simulink model "ARDRONE_SIM"  (R2014b)
settings: Solver=ode45  StartTime=0.0  StopTime=10  FixedStep=1/400  MaxStep=1  RelTol=1e-3
undefined symbols (not defined in the file or in its folder): X, Y, Z
libraries: sm_lib x204, fl_lib x82, nesl_utility x13, elec_lib x12, simulink x5, aerolibtransform2 x2, aerolibconvert2 x1
(part 2 of 5)

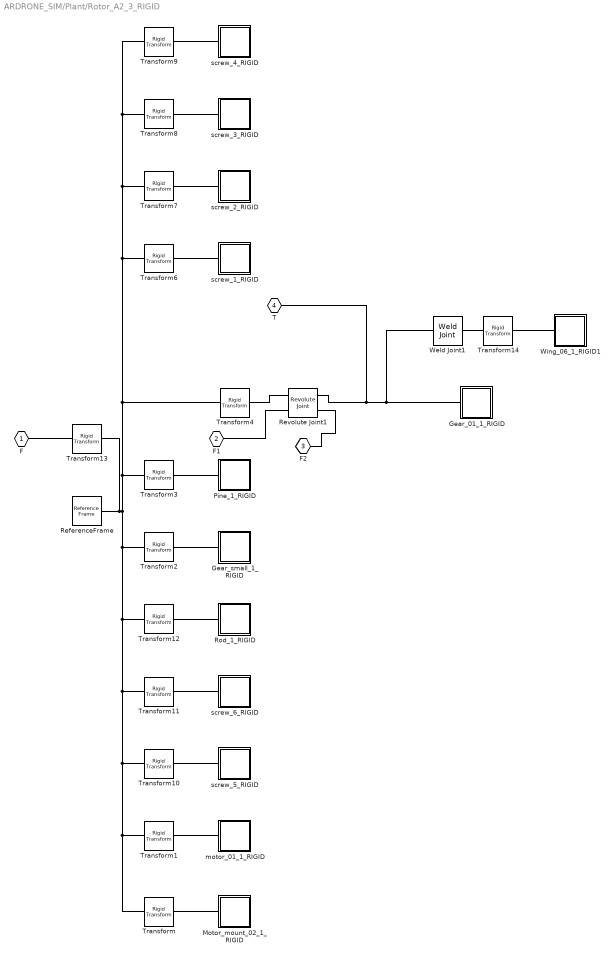
== system ARDRONE_SIM/Plant/Rotor_A2_3_RIGID ==
  Gear_01_1_RIGID : Subsystem
  Gear_small_1_RIGID : Subsystem
  Motor_mount_02_1_RIGID : Subsystem
  Pine_1_RIGID : Subsystem
  ReferenceFrame : sm_lib/Frames and Transforms/Reference Frame  BlockFunction=simmechanics.library.frames_transforms.reference_frame
  Revolute Joint1 : sm_lib/Joints/Revolute Joint  SenseConstraintForce=off  SenseConstraintForceX=off  SenseConstraintForceY=off  SenseConstraintForceZ=off  SenseConstraintTorque=off  SenseConstraintTorqueX=off  SenseConstraintTorqueY=off  SenseConstraintTorqueZ=off  SenseTotalForce=off  SenseTotalForceX=off  SenseTotalForceY=off  SenseTotalForceZ=off  SenseTotalTorque=off  SenseTotalTorqueX=off  SenseTotalTorqueY=off  SenseTotalTorqueZ=off  CompositeWrenchDir=FollowerOnBase  CompositeWrenchFrame=BaseFrame  EquilibriumPosition=0  EquilibriumPositionUnits=deg  SpringStiffness=0  SpringStiffnessUnits=N*m/deg  DampingCoefficient=0  DampingCoefficientUnits=N*m/(deg/s)  TorqueActuationMode=InputTorque  MotionActuationMode=ComputedMotion  SensePosition=off  SenseVelocity=on  SenseAcceleration=off  SenseTorqueForce=off  PositionTargetValue=0  PositionTargetValueUnits=deg  PositionTargetSpecify=off  PositionTargetPriority=High  VelocityTargetValue=500  VelocityTargetValueUnits=deg/s  VelocityTargetSpecify=off  VelocityTargetPriority=High  BlockFunction=simmechanics.library.joints.revolute_joint
  Rod_1_RIGID : Subsystem
  Transform : sm_lib/Frames and Transforms/Rigid Transform  TranslationMethod=None  TranslationLengthUnit=m  TranslationStandardAxis=+Z  TranslationStandardOffset=0  TranslationCartesianOffset=[0 0 0]  TranslationROffset=0  TranslationROffsetUnits=m  TranslationZOffset=0  TranslationZOffsetUnits=m  TranslationThetaOffset=0  TranslationThetaOffsetUnits=deg  RotationMethod=None  RotationAngleUnits=deg  RotationStandardAxis=+Z  RotationAngle=0  RotationArbitraryAxis=[0 0 1]  FollAlignAxisA=+X  BaseAlignAxisA=+Y  FollAlignAxisB=+Y  BaseAlignAxisB=+Z  RotationMatrix=[1 0 0; 0 1 0; 0 0 1]  BlockFunction=simmechanics.library.frames_transforms.rigid_transform
  Transform1 : sm_lib/Frames and Transforms/Rigid Transform  TranslationMethod=Cartesian  TranslationLengthUnit=mm  TranslationStandardAxis=+Z  TranslationStandardOffset=0  TranslationCartesianOffset=[3.1499999999999999 0 -20.598100000000002]  TranslationROffset=0  TranslationROffsetUnits=m  TranslationZOffset=0  TranslationZOffsetUnits=m  TranslationThetaOffset=0  TranslationThetaOffsetUnits=deg  RotationMethod=ArbitraryAxis  RotationAngleUnits=rad  RotationStandardAxis=+Z  RotationAngle=3.1403990331346985  RotationArbitraryAxis=[0 0 1]  FollAlignAxisA=+X  BaseAlignAxisA=+Y  FollAlignAxisB=+Y  BaseAlignAxisB=+Z  RotationMatrix=[1 0 0; 0 1 0; 0 0 1]  BlockFunction=simmechanics.library.frames_transforms.rigid_transform
  Transform10 : sm_lib/Frames and Transforms/Rigid Transform  TranslationMethod=Cartesian  TranslationLengthUnit=mm  TranslationStandardAxis=+Z  TranslationStandardOffset=0  TranslationCartesianOffset=[-19.174799999999998 6.3336399999999999 -3.4415300000000002]  TranslationROffset=0  TranslationROffsetUnits=m  TranslationZOffset=0  TranslationZOffsetUnits=m  TranslationThetaOffset=0  TranslationThetaOffsetUnits=deg  RotationMethod=ArbitraryAxis  RotationAngleUnits=rad  RotationStandardAxis=+Z  RotationAngle=1.5707963267948968  RotationArbitraryAxis=[0 1 0]  FollAlignAxisA=+X  BaseAlignAxisA=+Y  FollAlignAxisB=+Y  BaseAlignAxisB=+Z  RotationMatrix=[1 0 0; 0 1 0; 0 0 1]  BlockFunction=simmechanics.library.frames_transforms.rigid_transform
  Transform11 : sm_lib/Frames and Transforms/Rigid Transform  TranslationMethod=Cartesian  TranslationLengthUnit=mm  TranslationStandardAxis=+Z  TranslationStandardOffset=0  TranslationCartesianOffset=[21.5288 3.5415400000000004 -3.4415300000000002]  TranslationROffset=0  TranslationROffsetUnits=m  TranslationZOffset=0  TranslationZOffsetUnits=m  TranslationThetaOffset=0  TranslationThetaOffsetUnits=deg  RotationMethod=ArbitraryAxis  RotationAngleUnits=rad  RotationStandardAxis=+Z  RotationAngle=1.5707963267948968  RotationArbitraryAxis=[0 1 0]  FollAlignAxisA=+X  BaseAlignAxisA=+Y  FollAlignAxisB=+Y  BaseAlignAxisB=+Z  RotationMatrix=[1 0 0; 0 1 0; 0 0 1]  BlockFunction=simmechanics.library.frames_transforms.rigid_transform
  Transform12 : sm_lib/Frames and Transforms/Rigid Transform  TranslationMethod=Cartesian  TranslationLengthUnit=mm  TranslationStandardAxis=+Z  TranslationStandardOffset=0  TranslationCartesianOffset=[-18.649999999999999 0.033281699999999997 4.0656299999999996]  TranslationROffset=0  TranslationROffsetUnits=m  TranslationZOffset=0  TranslationZOffsetUnits=m  TranslationThetaOffset=0  TranslationThetaOffsetUnits=deg  RotationMethod=ArbitraryAxis  RotationAngleUnits=rad  RotationStandardAxis=+Z  RotationAngle=2.0943951023931953  RotationArbitraryAxis=[0.57735026918962584 -0.57735026918962584 -0.57735026918962584]  FollAlignAxisA=+X  BaseAlignAxisA=+Y  FollAlignAxisB=+Y  BaseAlignAxisB=+Z  RotationMatrix=[1 0 0; 0 1 0; 0 0 1]  BlockFunction=simmechanics.library.frames_transforms.rigid_transform
  Transform13 : sm_lib/Frames and Transforms/Rigid Transform  TranslationMethod=Cartesian  TranslationLengthUnit=mm  TranslationStandardAxis=+Z  TranslationStandardOffset=0  TranslationCartesianOffset=[0.036458000000000004 158.29999999999998 -8.3114100000000004]  TranslationROffset=0  TranslationROffsetUnits=m  TranslationZOffset=0  TranslationZOffsetUnits=m  TranslationThetaOffset=0  TranslationThetaOffsetUnits=deg  RotationMethod=ArbitraryAxis  RotationAngleUnits=rad  RotationStandardAxis=+Z  RotationAngle=1.5707964793812017  RotationArbitraryAxis=[-0.00039062294039628431 -0.00039062294039628431 0.99999984741370684]  FollAlignAxisA=+X  BaseAlignAxisA=+Y  FollAlignAxisB=+Y  BaseAlignAxisB=+Z  RotationMatrix=[1 0 0; 0 1 0; 0 0 1]  BlockFunction=simmechanics.library.frames_transforms.rigid_transform
  Transform14 : sm_lib/Frames and Transforms/Rigid Transform  TranslationMethod=Cartesian  TranslationLengthUnit=mm  TranslationStandardAxis=+Z  TranslationStandardOffset=0  TranslationCartesianOffset=[-93.759200000000007+14 -6.75 19]  TranslationROffset=0  TranslationROffsetUnits=m  TranslationZOffset=0  TranslationZOffsetUnits=m  TranslationThetaOffset=0  TranslationThetaOffsetUnits=deg  RotationMethod=None  RotationAngleUnits=rad  RotationStandardAxis=+Z  RotationAngle=2.5698479866285431  RotationArbitraryAxis=[0 0 1]  FollAlignAxisA=+X  BaseAlignAxisA=+Y  FollAlignAxisB=+Y  BaseAlignAxisB=+Z  RotationMatrix=[1 0 0; 0 1 0; 0 0 1]  BlockFunction=simmechanics.library.frames_transforms.rigid_transform
  Transform2 : sm_lib/Frames and Transforms/Rigid Transform  TranslationMethod=Cartesian  TranslationLengthUnit=mm  TranslationStandardAxis=+Z  TranslationStandardOffset=0  TranslationCartesianOffset=[3.1499999999999999 0 16.5459]  TranslationROffset=0  TranslationROffsetUnits=m  TranslationZOffset=0  TranslationZOffsetUnits=m  TranslationThetaOffset=0  TranslationThetaOffsetUnits=deg  RotationMethod=ArbitraryAxis  RotationAngleUnits=rad  RotationStandardAxis=+Z  RotationAngle=2.5767486738905112  RotationArbitraryAxis=[0 0 1]  FollAlignAxisA=+X  BaseAlignAxisA=+Y  FollAlignAxisB=+Y  BaseAlignAxisB=+Z  RotationMatrix=[1 0 0; 0 1 0; 0 0 1]  BlockFunction=simmechanics.library.frames_transforms.rigid_transform
  Transform3 : sm_lib/Frames and Transforms/Rigid Transform  TranslationMethod=Cartesian  TranslationLengthUnit=mm  TranslationStandardAxis=+Z  TranslationStandardOffset=0  TranslationCartesianOffset=[23.150000000000002 0 16.899999999999999]  TranslationROffset=0  TranslationROffsetUnits=m  TranslationZOffset=0  TranslationZOffsetUnits=m  TranslationThetaOffset=0  TranslationThetaOffsetUnits=deg  RotationMethod=ArbitraryAxis  RotationAngleUnits=rad  RotationStandardAxis=+Z  RotationAngle=3.1415926535897931  RotationArbitraryAxis=[0.94291276431253201 0.33303981578258707 0]  FollAlignAxisA=+X  BaseAlignAxisA=+Y  FollAlignAxisB=+Y  BaseAlignAxisB=+Z  RotationMatrix=[1 0 0; 0 1 0; 0 0 1]  BlockFunction=simmechanics.library.frames_transforms.rigid_transform
  Transform4 : sm_lib/Frames and Transforms/Rigid Transform  TranslationMethod=Cartesian  TranslationLengthUnit=mm  TranslationStandardAxis=+Z  TranslationStandardOffset=0  TranslationCartesianOffset=[23.150000000000002 0 15.25]  TranslationROffset=0  TranslationROffsetUnits=m  TranslationZOffset=0  TranslationZOffsetUnits=m  TranslationThetaOffset=0  TranslationThetaOffsetUnits=deg  RotationMethod=ArbitraryAxis  RotationAngleUnits=rad  RotationStandardAxis=+Z  RotationAngle=2.5698479866285431  RotationArbitraryAxis=[0 0 1]  FollAlignAxisA=+X  BaseAlignAxisA=+Y  FollAlignAxisB=+Y  BaseAlignAxisB=+Z  RotationMatrix=[1 0 0; 0 1 0; 0 0 1]  BlockFunction=simmechanics.library.frames_transforms.rigid_transform
  Transform6 : sm_lib/Frames and Transforms/Rigid Transform  TranslationMethod=Cartesian  TranslationLengthUnit=mm  TranslationStandardAxis=+Z  TranslationStandardOffset=0  TranslationCartesianOffset=[0.86552300000000004 3.8769999999999998 8.9434500000000003]  TranslationROffset=0  TranslationROffsetUnits=m  TranslationZOffset=0  TranslationZOffsetUnits=m  TranslationThetaOffset=0  TranslationThetaOffsetUnits=deg  RotationMethod=ArbitraryAxis  RotationAngleUnits=rad  RotationStandardAxis=+Z  RotationAngle=1.6089415653150072  RotationArbitraryAxis=[0.19166392654548023 -0.96256422046652934 0.19166392654548023]  FollAlignAxisA=+X  BaseAlignAxisA=+Y  FollAlignAxisB=+Y  BaseAlignAxisB=+Z  RotationMatrix=[1 0 0; 0 1 0; 0 0 1]  BlockFunction=simmechanics.library.frames_transforms.rigid_transform
  Transform7 : sm_lib/Frames and Transforms/Rigid Transform  TranslationMethod=Cartesian  TranslationLengthUnit=mm  TranslationStandardAxis=+Z  TranslationStandardOffset=0  TranslationCartesianOffset=[0.9346540000000001 -3.9169199999999997 8.9434500000000003]  TranslationROffset=0  TranslationROffsetUnits=m  TranslationZOffset=0  TranslationZOffsetUnits=m  TranslationThetaOffset=0  TranslationThetaOffsetUnits=deg  RotationMethod=ArbitraryAxis  RotationAngleUnits=rad  RotationStandardAxis=+Z  RotationAngle=1.5707963267948968  RotationArbitraryAxis=[-0 -1 -0]  FollAlignAxisA=+X  BaseAlignAxisA=+Y  FollAlignAxisB=+Y  BaseAlignAxisB=+Z  RotationMatrix=[1 0 0; 0 1 0; 0 0 1]  BlockFunction=simmechanics.library.frames_transforms.rigid_transform
  Transform8 : sm_lib/Frames and Transforms/Rigid Transform  TranslationMethod=Cartesian  TranslationLengthUnit=mm  TranslationStandardAxis=+Z  TranslationStandardOffset=0  TranslationCartesianOffset=[7.6498200000000001 0.0399131 8.9434500000000003]  TranslationROffset=0  TranslationROffsetUnits=m  TranslationZOffset=0  TranslationZOffsetUnits=m  TranslationThetaOffset=0  TranslationThetaOffsetUnits=deg  RotationMethod=ArbitraryAxis  RotationAngleUnits=rad  RotationStandardAxis=+Z  RotationAngle=1.5707963267948968  RotationArbitraryAxis=[-0 -1 -0]  FollAlignAxisA=+X  BaseAlignAxisA=+Y  FollAlignAxisB=+Y  BaseAlignAxisB=+Z  RotationMatrix=[1 0 0; 0 1 0; 0 0 1]  BlockFunction=simmechanics.library.frames_transforms.rigid_transform
  Transform9 : sm_lib/Frames and Transforms/Rigid Transform  TranslationMethod=Cartesian  TranslationLengthUnit=mm  TranslationStandardAxis=+Z  TranslationStandardOffset=0  TranslationCartesianOffset=[-19.420099999999998 -6.4385499999999993 -3.4415300000000002]  TranslationROffset=0  TranslationROffsetUnits=m  TranslationZOffset=0  TranslationZOffsetUnits=m  TranslationThetaOffset=0  TranslationThetaOffsetUnits=deg  RotationMethod=ArbitraryAxis  RotationAngleUnits=rad  RotationStandardAxis=+Z  RotationAngle=1.5707963267948968  RotationArbitraryAxis=[0 1 0]  FollAlignAxisA=+X  BaseAlignAxisA=+Y  FollAlignAxisB=+Y  BaseAlignAxisB=+Z  RotationMatrix=[1 0 0; 0 1 0; 0 0 1]  BlockFunction=simmechanics.library.frames_transforms.rigid_transform
  Weld Joint1 : sm_lib/Joints/Weld Joint  SenseConstraintForce=off  SenseConstraintForceX=off  SenseConstraintForceY=off  SenseConstraintForceZ=off  SenseConstraintTorque=off  SenseConstraintTorqueX=off  SenseConstraintTorqueY=off  SenseConstraintTorqueZ=off  SenseTotalForce=off  SenseTotalForceX=off  SenseTotalForceY=off  SenseTotalForceZ=off  SenseTotalTorque=off  SenseTotalTorqueX=off  SenseTotalTorqueY=off  SenseTotalTorqueZ=off  CompositeWrenchDir=FollowerOnBase  CompositeWrenchFrame=BaseFrame  BlockFunction=simmechanics.library.joints.weld_joint
  Wing_06_1_RIGID1 : Subsystem
  motor_01_1_RIGID : Subsystem
  screw_1_RIGID : Subsystem
  screw_2_RIGID : Subsystem
  screw_3_RIGID : Subsystem
  screw_4_RIGID : Subsystem
  screw_5_RIGID : Subsystem
  screw_6_RIGID : Subsystem
  F : PMIOPort  Port=1  Side=Left
  F1 : PMIOPort  Port=2  Side=Right
  F2 : PMIOPort  Port=3  Side=Left
  T : PMIOPort  Port=4  Side=Right
  connections:
  Motor_mount_02_1_RIGID/LConn1 -- Transform/RConn1
  Transform1/RConn1 -- motor_01_1_RIGID/LConn1
  Transform10/RConn1 -- screw_5_RIGID/LConn1
  Transform11/RConn1 -- screw_6_RIGID/LConn1
  Rod_1_RIGID/LConn1 -- Transform12/RConn1
  Transform13/LConn1 -- F/RConn1
  Gear_small_1_RIGID/LConn1 -- Transform2/RConn1
  Pine_1_RIGID/LConn1 -- Transform3/RConn1
  Transform6/RConn1 -- screw_1_RIGID/LConn1
  Transform7/RConn1 -- screw_2_RIGID/LConn1
  Transform8/RConn1 -- screw_3_RIGID/LConn1
  Transform9/RConn1 -- screw_4_RIGID/LConn1
  Weld Joint1/LConn1 -- T/RConn1 -- Revolute Joint1/RConn1 -- Gear_01_1_RIGID/LConn1
  Transform14/RConn1 -- Wing_06_1_RIGID1/LConn1
  Transform/LConn1 -- Transform4/LConn1 -- Transform8/LConn1 -- Transform9/LConn1 -- Transform7/LConn1 -- Transform6/LConn1 -- Transform3/LConn1 -- ReferenceFrame/RConn1 -- Transform13/RConn1 -- Transform2/LConn1 -- Transform12/LConn1 -- Transform11/LConn1 -- Transform10/LConn1 -- Transform1/LConn1
  Transform14/LConn1 -- Weld Joint1/RConn1
  Transform4/RConn1 -- Revolute Joint1/LConn1
  F1/RConn1 -- Revolute Joint1/LConn2
  F2/RConn1 -- Revolute Joint1/RConn2

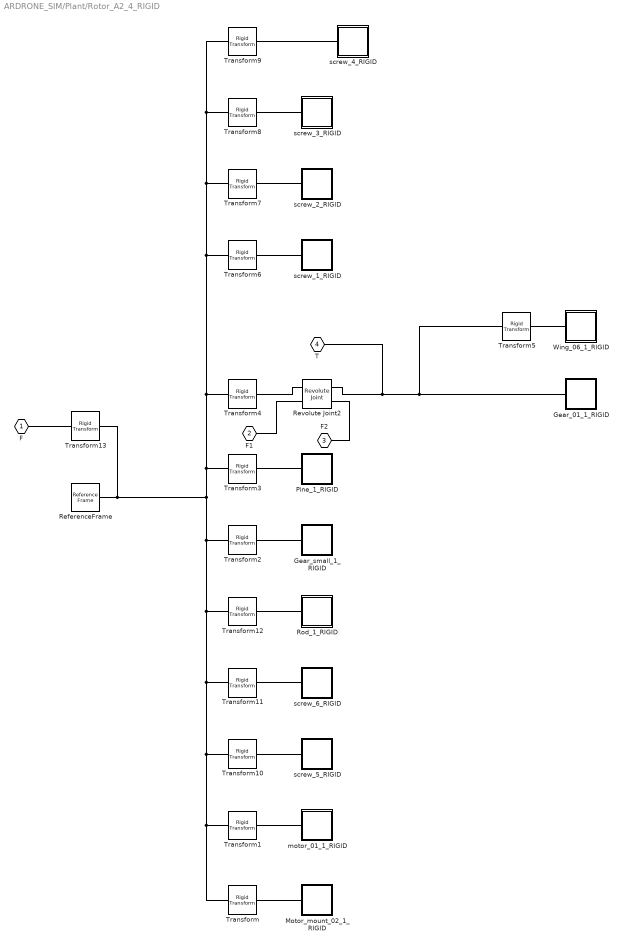
== system ARDRONE_SIM/Plant/Rotor_A2_4_RIGID ==
  Gear_01_1_RIGID : Subsystem
  Gear_small_1_RIGID : Subsystem
  Motor_mount_02_1_RIGID : Subsystem
  Pine_1_RIGID : Subsystem
  ReferenceFrame : sm_lib/Frames and Transforms/Reference Frame  BlockFunction=simmechanics.library.frames_transforms.reference_frame
  Revolute Joint2 : sm_lib/Joints/Revolute Joint  SenseConstraintForce=off  SenseConstraintForceX=off  SenseConstraintForceY=off  SenseConstraintForceZ=off  SenseConstraintTorque=off  SenseConstraintTorqueX=off  SenseConstraintTorqueY=off  SenseConstraintTorqueZ=off  SenseTotalForce=off  SenseTotalForceX=off  SenseTotalForceY=off  SenseTotalForceZ=off  SenseTotalTorque=off  SenseTotalTorqueX=off  SenseTotalTorqueY=off  SenseTotalTorqueZ=off  CompositeWrenchDir=FollowerOnBase  CompositeWrenchFrame=BaseFrame  EquilibriumPosition=0  EquilibriumPositionUnits=deg  SpringStiffness=0  SpringStiffnessUnits=N*m/deg  DampingCoefficient=0  DampingCoefficientUnits=N*m/(deg/s)  TorqueActuationMode=InputTorque  MotionActuationMode=ComputedMotion  SensePosition=off  SenseVelocity=on  SenseAcceleration=off  SenseTorqueForce=off  PositionTargetValue=0  PositionTargetValueUnits=deg  PositionTargetSpecify=off  PositionTargetPriority=High  VelocityTargetValue=500  VelocityTargetValueUnits=deg/s  VelocityTargetSpecify=off  VelocityTargetPriority=High  BlockFunction=simmechanics.library.joints.revolute_joint
  Rod_1_RIGID : Subsystem
  Transform : sm_lib/Frames and Transforms/Rigid Transform  TranslationMethod=None  TranslationLengthUnit=m  TranslationStandardAxis=+Z  TranslationStandardOffset=0  TranslationCartesianOffset=[0 0 0]  TranslationROffset=0  TranslationROffsetUnits=m  TranslationZOffset=0  TranslationZOffsetUnits=m  TranslationThetaOffset=0  TranslationThetaOffsetUnits=deg  RotationMethod=None  RotationAngleUnits=deg  RotationStandardAxis=+Z  RotationAngle=0  RotationArbitraryAxis=[0 0 1]  FollAlignAxisA=+X  BaseAlignAxisA=+Y  FollAlignAxisB=+Y  BaseAlignAxisB=+Z  RotationMatrix=[1 0 0; 0 1 0; 0 0 1]  BlockFunction=simmechanics.library.frames_transforms.rigid_transform
  Transform1 : sm_lib/Frames and Transforms/Rigid Transform  TranslationMethod=Cartesian  TranslationLengthUnit=mm  TranslationStandardAxis=+Z  TranslationStandardOffset=0  TranslationCartesianOffset=[3.1499999999999999 0 -20.598100000000002]  TranslationROffset=0  TranslationROffsetUnits=m  TranslationZOffset=0  TranslationZOffsetUnits=m  TranslationThetaOffset=0  TranslationThetaOffsetUnits=deg  RotationMethod=ArbitraryAxis  RotationAngleUnits=rad  RotationStandardAxis=+Z  RotationAngle=3.1403990331346985  RotationArbitraryAxis=[0 0 1]  FollAlignAxisA=+X  BaseAlignAxisA=+Y  FollAlignAxisB=+Y  BaseAlignAxisB=+Z  RotationMatrix=[1 0 0; 0 1 0; 0 0 1]  BlockFunction=simmechanics.library.frames_transforms.rigid_transform
  Transform10 : sm_lib/Frames and Transforms/Rigid Transform  TranslationMethod=Cartesian  TranslationLengthUnit=mm  TranslationStandardAxis=+Z  TranslationStandardOffset=0  TranslationCartesianOffset=[-19.174799999999998 6.3336399999999999 -3.4415300000000002]  TranslationROffset=0  TranslationROffsetUnits=m  TranslationZOffset=0  TranslationZOffsetUnits=m  TranslationThetaOffset=0  TranslationThetaOffsetUnits=deg  RotationMethod=ArbitraryAxis  RotationAngleUnits=rad  RotationStandardAxis=+Z  RotationAngle=1.5707963267948968  RotationArbitraryAxis=[0 1 0]  FollAlignAxisA=+X  BaseAlignAxisA=+Y  FollAlignAxisB=+Y  BaseAlignAxisB=+Z  RotationMatrix=[1 0 0; 0 1 0; 0 0 1]  BlockFunction=simmechanics.library.frames_transforms.rigid_transform
  Transform11 : sm_lib/Frames and Transforms/Rigid Transform  TranslationMethod=Cartesian  TranslationLengthUnit=mm  TranslationStandardAxis=+Z  TranslationStandardOffset=0  TranslationCartesianOffset=[21.5288 3.5415400000000004 -3.4415300000000002]  TranslationROffset=0  TranslationROffsetUnits=m  TranslationZOffset=0  TranslationZOffsetUnits=m  TranslationThetaOffset=0  TranslationThetaOffsetUnits=deg  RotationMethod=ArbitraryAxis  RotationAngleUnits=rad  RotationStandardAxis=+Z  RotationAngle=1.5707963267948968  RotationArbitraryAxis=[0 1 0]  FollAlignAxisA=+X  BaseAlignAxisA=+Y  FollAlignAxisB=+Y  BaseAlignAxisB=+Z  RotationMatrix=[1 0 0; 0 1 0; 0 0 1]  BlockFunction=simmechanics.library.frames_transforms.rigid_transform
  Transform12 : sm_lib/Frames and Transforms/Rigid Transform  TranslationMethod=Cartesian  TranslationLengthUnit=mm  TranslationStandardAxis=+Z  TranslationStandardOffset=0  TranslationCartesianOffset=[-18.649999999999999 0.033281699999999997 4.0656299999999996]  TranslationROffset=0  TranslationROffsetUnits=m  TranslationZOffset=0  TranslationZOffsetUnits=m  TranslationThetaOffset=0  TranslationThetaOffsetUnits=deg  RotationMethod=ArbitraryAxis  RotationAngleUnits=rad  RotationStandardAxis=+Z  RotationAngle=2.0943951023931953  RotationArbitraryAxis=[0.57735026918962584 -0.57735026918962584 -0.57735026918962584]  FollAlignAxisA=+X  BaseAlignAxisA=+Y  FollAlignAxisB=+Y  BaseAlignAxisB=+Z  RotationMatrix=[1 0 0; 0 1 0; 0 0 1]  BlockFunction=simmechanics.library.frames_transforms.rigid_transform
  Transform13 : sm_lib/Frames and Transforms/Rigid Transform  TranslationMethod=Cartesian  TranslationLengthUnit=mm  TranslationStandardAxis=+Z  TranslationStandardOffset=0  TranslationCartesianOffset=[158.29999999999998 -0.037259299999999995 -8.3156300000000005]  TranslationROffset=0  TranslationROffsetUnits=m  TranslationZOffset=0  TranslationZOffsetUnits=m  TranslationThetaOffset=0  TranslationThetaOffsetUnits=deg  RotationMethod=None  RotationAngleUnits=deg  RotationStandardAxis=+Z  RotationAngle=0  RotationArbitraryAxis=[0 0 1]  FollAlignAxisA=+X  BaseAlignAxisA=+Y  FollAlignAxisB=+Y  BaseAlignAxisB=+Z  RotationMatrix=[1 0 0; 0 1 0; 0 0 1]  BlockFunction=simmechanics.library.frames_transforms.rigid_transform
  Transform2 : sm_lib/Frames and Transforms/Rigid Transform  TranslationMethod=Cartesian  TranslationLengthUnit=mm  TranslationStandardAxis=+Z  TranslationStandardOffset=0  TranslationCartesianOffset=[3.1499999999999999 0 16.5459]  TranslationROffset=0  TranslationROffsetUnits=m  TranslationZOffset=0  TranslationZOffsetUnits=m  TranslationThetaOffset=0  TranslationThetaOffsetUnits=deg  RotationMethod=ArbitraryAxis  RotationAngleUnits=rad  RotationStandardAxis=+Z  RotationAngle=2.5767486738905112  RotationArbitraryAxis=[0 0 1]  FollAlignAxisA=+X  BaseAlignAxisA=+Y  FollAlignAxisB=+Y  BaseAlignAxisB=+Z  RotationMatrix=[1 0 0; 0 1 0; 0 0 1]  BlockFunction=simmechanics.library.frames_transforms.rigid_transform
  Transform3 : sm_lib/Frames and Transforms/Rigid Transform  TranslationMethod=Cartesian  TranslationLengthUnit=mm  TranslationStandardAxis=+Z  TranslationStandardOffset=0  TranslationCartesianOffset=[23.150000000000002 0 16.899999999999999]  TranslationROffset=0  TranslationROffsetUnits=m  TranslationZOffset=0  TranslationZOffsetUnits=m  TranslationThetaOffset=0  TranslationThetaOffsetUnits=deg  RotationMethod=ArbitraryAxis  RotationAngleUnits=rad  RotationStandardAxis=+Z  RotationAngle=3.1415926535897931  RotationArbitraryAxis=[0.94291276431253201 0.33303981578258707 0]  FollAlignAxisA=+X  BaseAlignAxisA=+Y  FollAlignAxisB=+Y  BaseAlignAxisB=+Z  RotationMatrix=[1 0 0; 0 1 0; 0 0 1]  BlockFunction=simmechanics.library.frames_transforms.rigid_transform
  Transform4 : sm_lib/Frames and Transforms/Rigid Transform  TranslationMethod=Cartesian  TranslationLengthUnit=mm  TranslationStandardAxis=+Z  TranslationStandardOffset=0  TranslationCartesianOffset=[23.150000000000002 0 15.25]  TranslationROffset=0  TranslationROffsetUnits=m  TranslationZOffset=0  TranslationZOffsetUnits=m  TranslationThetaOffset=0  TranslationThetaOffsetUnits=deg  RotationMethod=ArbitraryAxis  RotationAngleUnits=rad  RotationStandardAxis=+Z  RotationAngle=2.5698479866285431  RotationArbitraryAxis=[0 0 1]  FollAlignAxisA=+X  BaseAlignAxisA=+Y  FollAlignAxisB=+Y  BaseAlignAxisB=+Z  RotationMatrix=[1 0 0; 0 1 0; 0 0 1]  BlockFunction=simmechanics.library.frames_transforms.rigid_transform
  Transform5 : sm_lib/Frames and Transforms/Rigid Transform  TranslationMethod=Cartesian  TranslationLengthUnit=mm  TranslationStandardAxis=+Z  TranslationStandardOffset=0  TranslationCartesianOffset=[-93.759200000000007+14 -6.75 19]  TranslationROffset=0  TranslationROffsetUnits=m  TranslationZOffset=0  TranslationZOffsetUnits=m  TranslationThetaOffset=0  TranslationThetaOffsetUnits=deg  RotationMethod=None  RotationAngleUnits=rad  RotationStandardAxis=+Z  RotationAngle=2.5698479866285431  RotationArbitraryAxis=[0 0 1]  FollAlignAxisA=+X  BaseAlignAxisA=+Y  FollAlignAxisB=+Y  BaseAlignAxisB=+Z  RotationMatrix=[1 0 0; 0 1 0; 0 0 1]  BlockFunction=simmechanics.library.frames_transforms.rigid_transform
  Transform6 : sm_lib/Frames and Transforms/Rigid Transform  TranslationMethod=Cartesian  TranslationLengthUnit=mm  TranslationStandardAxis=+Z  TranslationStandardOffset=0  TranslationCartesianOffset=[0.86552300000000004 3.8769999999999998 8.9434500000000003]  TranslationROffset=0  TranslationROffsetUnits=m  TranslationZOffset=0  TranslationZOffsetUnits=m  TranslationThetaOffset=0  TranslationThetaOffsetUnits=deg  RotationMethod=ArbitraryAxis  RotationAngleUnits=rad  RotationStandardAxis=+Z  RotationAngle=1.6089415653150072  RotationArbitraryAxis=[0.19166392654548023 -0.96256422046652934 0.19166392654548023]  FollAlignAxisA=+X  BaseAlignAxisA=+Y  FollAlignAxisB=+Y  BaseAlignAxisB=+Z  RotationMatrix=[1 0 0; 0 1 0; 0 0 1]  BlockFunction=simmechanics.library.frames_transforms.rigid_transform
  Transform7 : sm_lib/Frames and Transforms/Rigid Transform  TranslationMethod=Cartesian  TranslationLengthUnit=mm  TranslationStandardAxis=+Z  TranslationStandardOffset=0  TranslationCartesianOffset=[0.9346540000000001 -3.9169199999999997 8.9434500000000003]  TranslationROffset=0  TranslationROffsetUnits=m  TranslationZOffset=0  TranslationZOffsetUnits=m  TranslationThetaOffset=0  TranslationThetaOffsetUnits=deg  RotationMethod=ArbitraryAxis  RotationAngleUnits=rad  RotationStandardAxis=+Z  RotationAngle=1.5707963267948968  RotationArbitraryAxis=[-0 -1 -0]  FollAlignAxisA=+X  BaseAlignAxisA=+Y  FollAlignAxisB=+Y  BaseAlignAxisB=+Z  RotationMatrix=[1 0 0; 0 1 0; 0 0 1]  BlockFunction=simmechanics.library.frames_transforms.rigid_transform
  Transform8 : sm_lib/Frames and Transforms/Rigid Transform  TranslationMethod=Cartesian  TranslationLengthUnit=mm  TranslationStandardAxis=+Z  TranslationStandardOffset=0  TranslationCartesianOffset=[7.6498200000000001 0.0399131 8.9434500000000003]  TranslationROffset=0  TranslationROffsetUnits=m  TranslationZOffset=0  TranslationZOffsetUnits=m  TranslationThetaOffset=0  TranslationThetaOffsetUnits=deg  RotationMethod=ArbitraryAxis  RotationAngleUnits=rad  RotationStandardAxis=+Z  RotationAngle=1.5707963267948968  RotationArbitraryAxis=[-0 -1 -0]  FollAlignAxisA=+X  BaseAlignAxisA=+Y  FollAlignAxisB=+Y  BaseAlignAxisB=+Z  RotationMatrix=[1 0 0; 0 1 0; 0 0 1]  BlockFunction=simmechanics.library.frames_transforms.rigid_transform
  Transform9 : sm_lib/Frames and Transforms/Rigid Transform  TranslationMethod=Cartesian  TranslationLengthUnit=mm  TranslationStandardAxis=+Z  TranslationStandardOffset=0  TranslationCartesianOffset=[-19.420099999999998 -6.4385499999999993 -3.4415300000000002]  TranslationROffset=0  TranslationROffsetUnits=m  TranslationZOffset=0  TranslationZOffsetUnits=m  TranslationThetaOffset=0  TranslationThetaOffsetUnits=deg  RotationMethod=ArbitraryAxis  RotationAngleUnits=rad  RotationStandardAxis=+Z  RotationAngle=1.5707963267948968  RotationArbitraryAxis=[0 1 0]  FollAlignAxisA=+X  BaseAlignAxisA=+Y  FollAlignAxisB=+Y  BaseAlignAxisB=+Z  RotationMatrix=[1 0 0; 0 1 0; 0 0 1]  BlockFunction=simmechanics.library.frames_transforms.rigid_transform
  Wing_06_1_RIGID : Subsystem
  motor_01_1_RIGID : Subsystem
  screw_1_RIGID : Subsystem
  screw_2_RIGID : Subsystem
  screw_3_RIGID : Subsystem
  screw_4_RIGID : Subsystem
  screw_5_RIGID : Subsystem
  screw_6_RIGID : Subsystem
  F : PMIOPort  Port=1  Side=Left
  F1 : PMIOPort  Port=2  Side=Right
  F2 : PMIOPort  Port=3  Side=Left
  T : PMIOPort  Port=4  Side=Right
  connections:
  Motor_mount_02_1_RIGID/LConn1 -- Transform/RConn1
  Transform1/RConn1 -- motor_01_1_RIGID/LConn1
  Transform10/RConn1 -- screw_5_RIGID/LConn1
  Transform11/RConn1 -- screw_6_RIGID/LConn1
  Rod_1_RIGID/LConn1 -- Transform12/RConn1
  Transform13/LConn1 -- F/RConn1
  Gear_small_1_RIGID/LConn1 -- Transform2/RConn1
  Transform6/RConn1 -- screw_1_RIGID/LConn1
  Transform7/RConn1 -- screw_2_RIGID/LConn1
  Transform8/RConn1 -- screw_3_RIGID/LConn1
  Transform9/RConn1 -- screw_4_RIGID/LConn1
  Transform3/RConn1 -- Pine_1_RIGID/LConn1
  Gear_01_1_RIGID/LConn1 -- T/RConn1 -- Revolute Joint2/RConn1 -- Transform5/LConn1
  Transform5/RConn1 -- Wing_06_1_RIGID/LConn1
  ReferenceFrame/RConn1 -- Transform4/LConn1 -- Transform8/LConn1 -- Transform9/LConn1 -- Transform7/LConn1 -- Transform6/LConn1 -- Transform3/LConn1 -- Transform/LConn1 -- Transform1/LConn1 -- Transform10/LConn1 -- Transform11/LConn1 -- Transform12/LConn1 -- Transform2/LConn1 -- Transform13/RConn1
  Transform4/RConn1 -- Revolute Joint2/LConn1
  F1/RConn1 -- Revolute Joint2/LConn2
  Revolute Joint2/RConn2 -- F2/RConn1

== system ARDRONE_SIM/Plant/Subsystem ==
  Angular Velocity Source : fl_lib/Mechanical/Mechanical Sources/Ideal Angular Velocity Source
  Torque Sensor : fl_lib/Mechanical/Mechanical Sensors/Ideal Torque Sensor
  B : PMIOPort  Port=1  Side=Left
  F : PMIOPort  Port=2  Side=Left
  T2 : PMIOPort  Port=3  Side=Left
  T1 : PMIOPort  Port=4  Side=Right
  connections:
  T1/RConn1 -- Torque Sensor/RConn2
  T2/RConn1 -- Angular Velocity Source/RConn1
  Torque Sensor/LConn1 -- F/RConn1
  Angular Velocity Source/RConn2 -- B/RConn1
  Angular Velocity Source/LConn1 -- Torque Sensor/RConn1

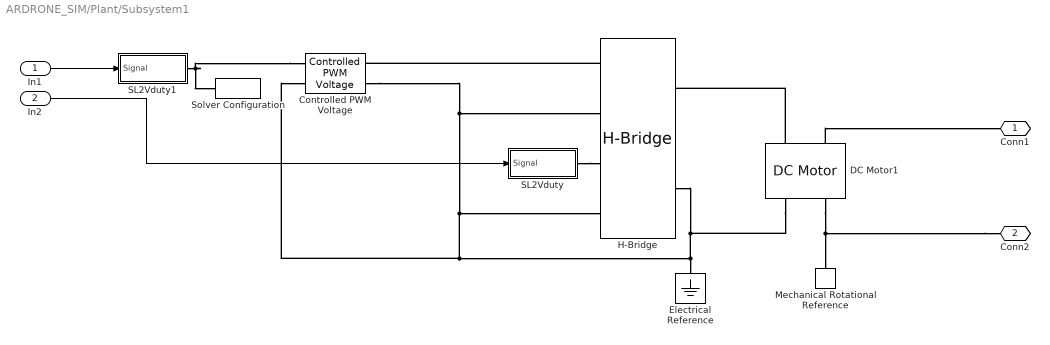
== system ARDRONE_SIM/Plant/Subsystem1 ==
  In1 : Inport
  In2 : Inport  Port=2
  Controlled PWM Voltage : elec_lib/Actuators & Drivers/Drivers/Controlled PWM Voltage  F=4000 Hz  TD=0 s  pulse_width_offset=0 s  Vmin=0 V  Vmax=100 V  Vm=5 V  pwm_or_av=2  event_type=1  sample_time=1e-6 s
  DC Motor1 : elec_lib/Actuators & Drivers/Rotational Actuators/DC Motor  parameterization=3  Ra=3.9 Ohm  La=0.01 H  emf_or_torque=1  Kv=7.2e-05 V/rpm  Ki=6.876e-04 N*m/A  T_stall=2.4e-04 N*m  w_max=5000 rpm  w_rated=4500 rpm  P_rated=15 W  V_rated=5 V  J=0.0002/4 kg*m^2  lam_param=1  lam=1e-06 N*m/(rad/s)  i_noload=0 A  V_i_noload=1.5 V  speed0=0 rpm  alpha=0.00393 1/K  Tmeas=25 C  thermal_mass=100 J/K  initial_temperature=25 C
  Electrical Reference : fl_lib/Electrical/Electrical Elements/Electrical Reference
  H-Bridge : elec_lib/Actuators & Drivers/Drivers/H-Bridge  Venable=2.5 V  Vmax=5 V  Vreverse=2.5 V  Vbrake=2.5 V  Vm=5 V  pwm_or_av=2  discontinuous=0  freewheeling_mode=1  freewheeling_mode_disc=1  Ron=0.01 Ohm  Don=0.1 Ohm  Rload=10 Ohm  Lload=1e-5 H  F=10 kHz  w_vec=[1, 2] s  i_vec=[1, 2] A  vMatrix=[1, 2; 3, 4] V
  Mechanical Rotational Reference : fl_lib/Mechanical/Rotational Elements/Mechanical Rotational Reference
  SL2Vduty : Subsystem
  SL2Vduty1 : Subsystem
  Solver Configuration : nesl_utility/Solver Configuration  PhysicalDomain=network_engine_domain  SubClassName=solver  LeftPortType=input  RightPortType=generic  Accelerate=off  Tones=[]  Harmonics=[]  SimulateNoise=off  Profile=off  UseLocalSampling=off  EnableSwitchedLinearOptims=on  FrequencyDomain=off  UseCCode=off  RelTol=0.001  AbsTol=1e-06  MinStep=1e-09  ToWorkspace=off  DoDC=off  ResidualTolerance=1e-9  UseLocalSolver=off  LocalSolverChoice=NE_BACKWARD_EULER_ADVANCER  LocalSolverSampleTime=.001  DoFixedCost=off  MaxNonlinIter=3  MaxModeIter=2  LinearAlgebra=Sparse  DelaysMemoryBudget=1024  AutomaticFiltering=on  FilteringTimeConstant=0.001
  Conn1 : PMIOPort  Port=1  Side=Right
  Conn2 : PMIOPort  Port=2  Side=Right
  wires:
  In1/1 -> SL2Vduty1/1(Signal)
  In2/1 -> SL2Vduty/1(Signal)
  connections:
  DC Motor1/LConn2 -- Conn1/RConn1
  Controlled PWM Voltage/LConn1 -- Solver Configuration/RConn1 -- SL2Vduty1/RConn1
  Conn2/RConn1 -- DC Motor1/RConn2 -- Mechanical Rotational Reference/LConn1
  H-Bridge/LConn1 -- Controlled PWM Voltage/RConn1
  Controlled PWM Voltage/LConn2 -- H-Bridge/LConn2 -- Controlled PWM Voltage/RConn2 -- H-Bridge/LConn4 -- Electrical Reference/LConn1 -- DC Motor1/RConn1 -- H-Bridge/RConn2
  SL2Vduty/RConn1 -- H-Bridge/LConn3
  DC Motor1/LConn1 -- H-Bridge/RConn1

== system ARDRONE_SIM/Plant/Subsystem2 ==
  Angular Velocity Source : fl_lib/Mechanical/Mechanical Sources/Ideal Angular Velocity Source
  Torque Sensor : fl_lib/Mechanical/Mechanical Sensors/Ideal Torque Sensor
  B : PMIOPort  Port=1  Side=Left
  F : PMIOPort  Port=2  Side=Left
  T2 : PMIOPort  Port=3  Side=Left
  T1 : PMIOPort  Port=4  Side=Right
  connections:
  Angular Velocity Source/LConn1 -- Torque Sensor/RConn1
  Angular Velocity Source/RConn2 -- B/RConn1
  Torque Sensor/LConn1 -- F/RConn1
  T2/RConn1 -- Angular Velocity Source/RConn1
  T1/RConn1 -- Torque Sensor/RConn2

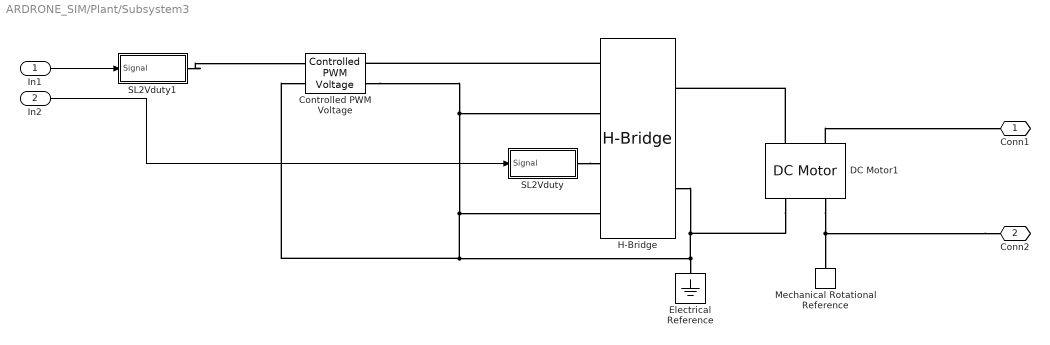
== system ARDRONE_SIM/Plant/Subsystem3 ==
  In1 : Inport
  In2 : Inport  Port=2
  Controlled PWM Voltage : elec_lib/Actuators & Drivers/Drivers/Controlled PWM Voltage  F=4000 Hz  TD=0 s  pulse_width_offset=0 s  Vmin=0 V  Vmax=100 V  Vm=5 V  pwm_or_av=2  event_type=1  sample_time=1e-6 s
  DC Motor1 : elec_lib/Actuators & Drivers/Rotational Actuators/DC Motor  parameterization=3  Ra=3.9 Ohm  La=0.01 H  emf_or_torque=1  Kv=7.2e-05 V/rpm  Ki=6.876e-04 N*m/A  T_stall=2.4e-04 N*m  w_max=5000 rpm  w_rated=4500 rpm  P_rated=15 W  V_rated=5 V  J=0.0002/4 kg*m^2  lam_param=1  lam=1e-06 N*m/(rad/s)  i_noload=0 A  V_i_noload=1.5 V  speed0=0 rpm  alpha=0.00393 1/K  Tmeas=25 C  thermal_mass=100 J/K  initial_temperature=25 C
  Electrical Reference : fl_lib/Electrical/Electrical Elements/Electrical Reference
  H-Bridge : elec_lib/Actuators & Drivers/Drivers/H-Bridge  Venable=2.5 V  Vmax=5 V  Vreverse=2.5 V  Vbrake=2.5 V  Vm=5 V  pwm_or_av=2  discontinuous=0  freewheeling_mode=1  freewheeling_mode_disc=1  Ron=0.01 Ohm  Don=0.1 Ohm  Rload=10 Ohm  Lload=1e-5 H  F=10 kHz  w_vec=[1, 2] s  i_vec=[1, 2] A  vMatrix=[1, 2; 3, 4] V
  Mechanical Rotational Reference : fl_lib/Mechanical/Rotational Elements/Mechanical Rotational Reference
  SL2Vduty : Subsystem
  SL2Vduty1 : Subsystem
  Conn1 : PMIOPort  Port=1  Side=Right
  Conn2 : PMIOPort  Port=2  Side=Right
  wires:
  In2/1 -> SL2Vduty/1(Signal)
  In1/1 -> SL2Vduty1/1(Signal)
  connections:
  DC Motor1/LConn1 -- H-Bridge/RConn1
  SL2Vduty/RConn1 -- H-Bridge/LConn3
  H-Bridge/RConn2 -- DC Motor1/RConn1 -- Electrical Reference/LConn1 -- H-Bridge/LConn4 -- Controlled PWM Voltage/RConn2 -- H-Bridge/LConn2 -- Controlled PWM Voltage/LConn2
  H-Bridge/LConn1 -- Controlled PWM Voltage/RConn1
  Conn2/RConn1 -- DC Motor1/RConn2 -- Mechanical Rotational Reference/LConn1
  SL2Vduty1/RConn1 -- Controlled PWM Voltage/LConn1
  DC Motor1/LConn2 -- Conn1/RConn1
